simulink model "IMM_2model_turn_rate_Com"  (R2012b)
settings: Solver=FixedStepDiscrete  StartTime=0.0  StopTime=SimulStop  FixedStep=0.05  RelTol=1e-3
values from neighbouring files (symbols this model uses):
  A1 = [1 T 0 0;       0 1 0 0;       0 0 1 T;       0 0 0 1]    [parameter.m]
  A2 = [1 sin(r2*T)/r2 0 -(1-cos(r2*T))/r2;      0 cos(r2*T) 0 -sin(r2*T);      0 (1-cos(r2*T))/r2 1 sin(r2*T)/r2;      0 sin(r2*T) 0 cos(r2*T)]    [parameter.m]
  A3 = [1 T1 0 0;       0 1 0 0;       0 0 1 T1;       0 0 0 1]    [parameter.m]
  A4 = [1 sin(r2*T1)/r2 0 -(1-cos(r2*T1))/r2;      0 cos(r2*T1) 0 -sin(r2*T1);      0 (1-cos(r2*T1))/r2 1 sin(r2*T1)/r2;      0 sin(r2*T1) 0 cos(r2*T1)]    [parameter.m]
  C = [1 0 0 0; 0 0 1 0]    [parameter.m]
  mu1_init = 0.5    [parameter.m]
  mu2_init = 0.5    [parameter.m]
  P_init = eye(4)*5    [parameter.m]
  PHI = [0.99 0.01; 0.01 0.99]    [parameter.m]
  SimulStop = length(obv_traj1)*T    [parameter.m]
  T1 = 0.5    [parameter.m]
  V1 = Dw*Sv1*Dw'    [parameter.m]
  W1 = Bw*Sw1*Bw'    [parameter.m]
  W2 = Bw*Sw2*Bw'    [parameter.m]
  xhat_init = [obv_traj1(1,2);0 ;obv_traj1(1,3);0]    [parameter.m]
libraries: dspmtrx3 x10, dspinverses x2, commnoisgen2 x1
settings Model: Creator=DonghanLee  LastModifiedBy=DonghanLee

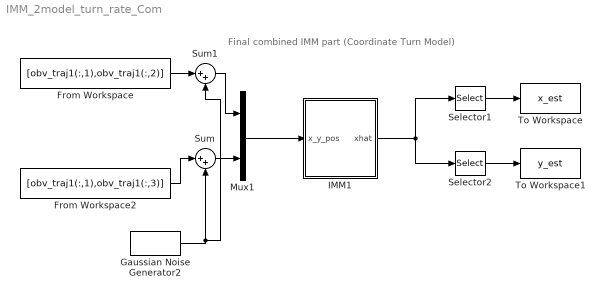
== system IMM_2model_turn_rate_Com ==
  note: Final combined IMM part (Coordinate Turn Model)
  From Workspace : FromWorkspace  VariableName=[obv_traj1(:,1),obv_traj1(:,2)]  SampleTime=0
  From Workspace2 : FromWorkspace  VariableName=[obv_traj1(:,1),obv_traj1(:,3)]  SampleTime=0
  Gaussian Noise Generator2 : commnoisgen2/Gaussian Noise Generator  m=0  d=noise  s=0  Ts=0.05  frameBased=off  sampPerFrame=1  orient=off  outDataType=double
  IMM1 : Subsystem
  Mux1 : Mux  Inputs=2
  Selector1 : Selector  InputPortWidth=4  IndexOptions=Index vector (dialog)  Indices=[1 2]  OutputSizes=1
  Selector2 : Selector  InputPortWidth=4  IndexOptions=Index vector (dialog)  Indices=[3 4]  OutputSizes=1
  Sum : Sum  Inputs=|++
  Sum1 : Sum  Inputs=|++
  To Workspace : ToWorkspace  VariableName=x_est  SampleTime=-1
  To Workspace1 : ToWorkspace  VariableName=y_est  SampleTime=-1
  wires:
  Mux1/1 -> IMM1/1(x_y_pos)
  Gaussian Noise Generator2/1 -> Sum1/2, Sum/2
  From Workspace2/1 -> Sum/1
  Sum/1 -> Mux1/2
  From Workspace/1 -> Sum1/1
  Sum1/1 -> Mux1/1
  IMM1/1(xhat) -> Selector2/1, Selector1/1
  Selector1/1 -> To Workspace/1
  Selector2/1 -> To Workspace1/1

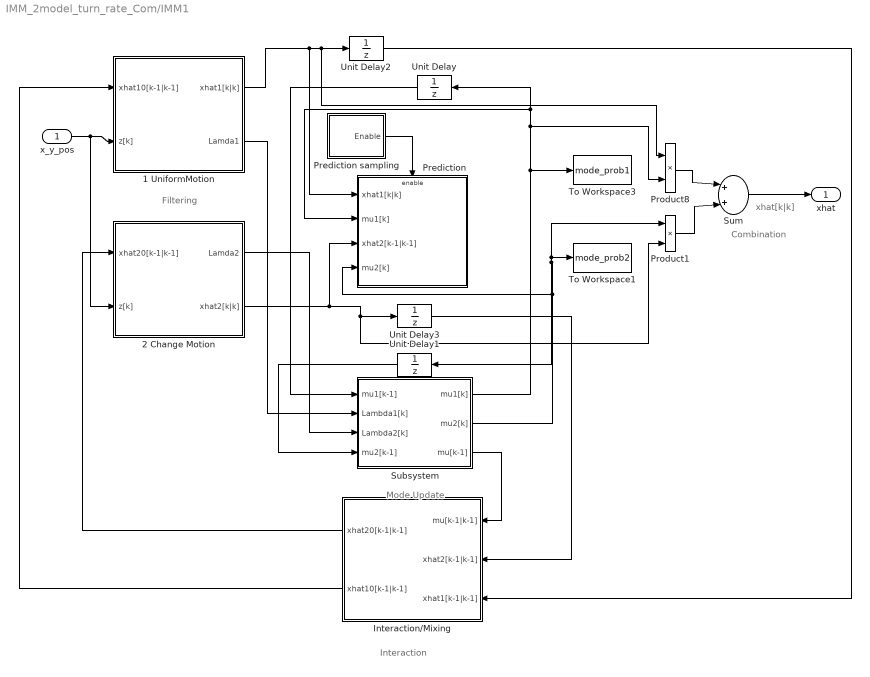
== system IMM_2model_turn_rate_Com/IMM1 ==
  note: Mode Update
  note: Interaction
  note: Filtering
  note: xhat[k|k]
  note: Combination
  x_y_pos : Inport
  "1 UniformMotion " : Subsystem
  "2 Change Motion " : Subsystem
  Interaction/Mixing : Subsystem
  Prediction : Subsystem
  Prediction sampling : Subsystem
  Product1 : Product  SaturateOnIntegerOverflow=on  OutDataTypeStr=Inherit: Same as first input
  Product8 : Product  SaturateOnIntegerOverflow=on  OutDataTypeStr=Inherit: Same as first input
  Subsystem : Subsystem
  Sum : Sum  Inputs=|++|  SaturateOnIntegerOverflow=on
  To Workspace1 : ToWorkspace  VariableName=mode_prob2  SampleTime=-1
  To Workspace3 : ToWorkspace  VariableName=mode_prob1  SampleTime=-1
  Unit Delay : UnitDelay  InitialCondition=mu1_init  SampleTime=-1
  Unit Delay1 : UnitDelay  InitialCondition=mu2_init  SampleTime=-1
  Unit Delay2 : UnitDelay  InitialCondition=xhat_init  SampleTime=-1
  Unit Delay3 : UnitDelay  InitialCondition=xhat_init  SampleTime=-1
  xhat : Outport
  wires:
  Product8/1 -> Sum/1
  Product1/1 -> Sum/2
  "2 Change Motion "/2(xhat2[k|k]) -> Prediction/3(xhat2[k-1|k-1]), Product1/2, Unit Delay3/1
  Subsystem/3(mu[k-1]) -> Interaction/Mixing/1(mu[k-1|k-1])
  Interaction/Mixing/1(xhat20[k-1|k-1]) -> "2 Change Motion "/1(xhat20[k-1|k-1])
  Interaction/Mixing/2(xhat10[k-1|k-1]) -> "1 UniformMotion "/1(xhat10[k-1|k-1])
  Sum/1 -> xhat/1
  Unit Delay/1 -> Subsystem/1(mu1[k-1])
  Unit Delay1/1 -> Subsystem/4(mu2[k-1])
  Unit Delay3/1 -> Interaction/Mixing/2(xhat2[k-1|k-1])
  Unit Delay2/1 -> Interaction/Mixing/3(xhat1[k-1|k-1])
  x_y_pos/1 -> "2 Change Motion "/2(z[k]), "1 UniformMotion "/2(z[k])
  "1 UniformMotion "/1(xhat1[k|k]) -> Prediction/1(xhat1[k|k]), Product8/1, Unit Delay2/1
  "1 UniformMotion "/2(Lamda1) -> Subsystem/2(Lambda1[k])
  "2 Change Motion "/1(Lamda2) -> Subsystem/3(Lambda2[k])
  Subsystem/1(mu1[k]) -> To Workspace3/1, Product8/2, Unit Delay/1, Prediction/2("mu1[k] ")
  Subsystem/2(mu2[k]) -> Product1/1, To Workspace1/1, Unit Delay1/1, Prediction/4(mu2[k])
  Prediction sampling/1(Enable) -> Prediction/Enable

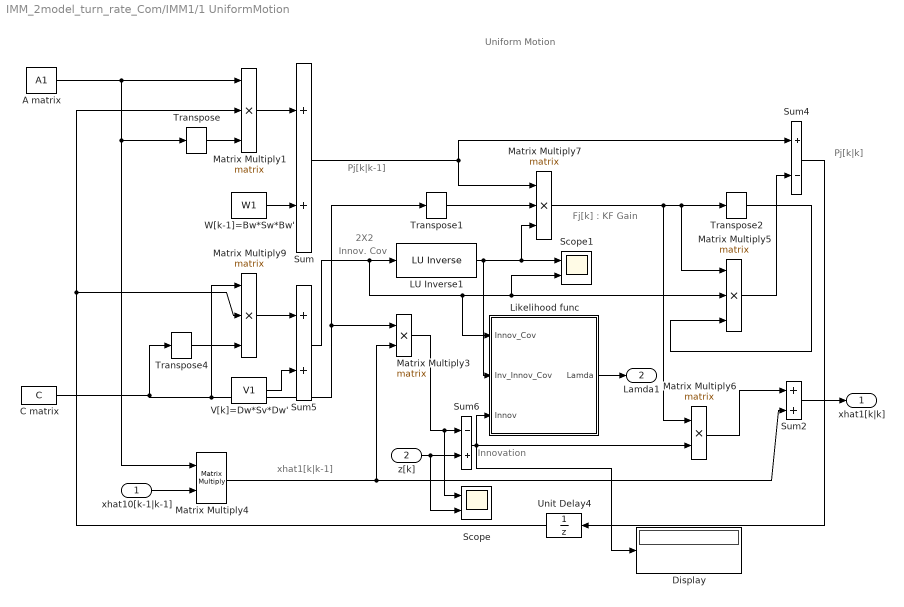
== system IMM_2model_turn_rate_Com/IMM1/1 UniformMotion  ==
  note: 2X2
  note: Pj[k|k]
  note: Innovation
  note: Innov. Cov
  note: Pj[k|k-1]
  note: xhat1[k|k-1]
  note: Uniform Motion
  note: Fj[k] : KF Gain
  xhat10[k-1|k-1] : Inport
  z[k] : Inport  Port=2
  " LU Inverse1" : dspinverses/ LU Inverse
  A matrix : Constant  Value=A1
  C matrix : Constant  Value=C
  Display : Display
  Likelihood func : Subsystem
  Matrix Multiply{1,5,7,9} (4 alike) : Product  Inputs=3  Multiplication=Matrix(*)
  Matrix Multiply3 : Product  Multiplication=Matrix(*)
  Matrix Multiply4 : Product  Multiplication=Matrix(*)
  Matrix Multiply6 : Product  Multiplication=Matrix(*)
  Scope : Scope  NumInputPorts=2
      settings: YMin=-5~5  YMax=5~20  SaveName=ScopeData10
  Scope1 : Scope  NumInputPorts=2
      settings: YMin=-0.00025~-5e+300  YMax=0.0015~3e+301  SaveName=ScopeData11
  Sum : Sum  SaturateOnIntegerOverflow=on
  Sum2 : Sum  SaturateOnIntegerOverflow=on
  Sum4 : Sum  Inputs=+-  SaturateOnIntegerOverflow=on
  Sum5 : Sum  SaturateOnIntegerOverflow=on
  Sum6 : Sum  Inputs=-+  SaturateOnIntegerOverflow=on
  Transpose{,1..2,4} (4 alike) : dspmtrx3/Transpose  Hermitian=off  overflowFlag=off
  Unit Delay4 : UnitDelay  InitialCondition=P_init  SampleTime=-1
  V[k]=Dw*Sv*Dw' : Constant  Value=V1
  "W[k-1]=Bw*Sw*Bw' " : Constant  Value=W1
  xhat1[k|k] : Outport
  Lamda1 : Outport  Port=2
  wires:
  Transpose/1 -> Matrix Multiply1/3
  A matrix/1 -> Matrix Multiply1/1, Matrix Multiply4/1, Transpose/1
  Matrix Multiply1/1 -> Sum/1
  Matrix Multiply3/1 -> Scope/1, Sum6/1
  C matrix/1 -> Transpose4/1, Matrix Multiply9/1, Transpose1/1, Matrix Multiply3/1
  Matrix Multiply4/1 -> Matrix Multiply3/2, Sum2/2
  Matrix Multiply7/1 -> Matrix Multiply6/1, Matrix Multiply5/1, Transpose2/1
  Transpose2/1 -> Matrix Multiply5/3
  Matrix Multiply6/1 -> Sum2/1
  Sum2/1 -> xhat1[k|k]/1
  "W[k-1]=Bw*Sw*Bw' "/1 -> Sum/2
  xhat10[k-1|k-1]/1 -> Matrix Multiply4/2
  Sum4/1 -> Unit Delay4/1
  Sum5/1 -> Likelihood func/1(Innov_Cov), Scope1/2, Matrix Multiply5/2, " LU Inverse1"/1
  " LU Inverse1"/1 -> Likelihood func/2(Inv_Innov_Cov), Scope1/1, Matrix Multiply7/3
  Unit Delay4/1 -> Matrix Multiply1/2, Matrix Multiply9/2
  Transpose4/1 -> Matrix Multiply9/3
  Matrix Multiply9/1 -> Sum5/1
  V[k]=Dw*Sv*Dw'/1 -> Sum5/2
  Transpose1/1 -> Matrix Multiply7/2
  z[k]/1 -> Scope/2, Sum6/2
  Sum6/1 -> Matrix Multiply6/2, Likelihood func/3(Innov), Display/1
  Matrix Multiply5/1 -> Sum4/2
  Sum/1 -> Sum4/1, Matrix Multiply7/1
  Likelihood func/1(Lamda) -> Lamda1/1

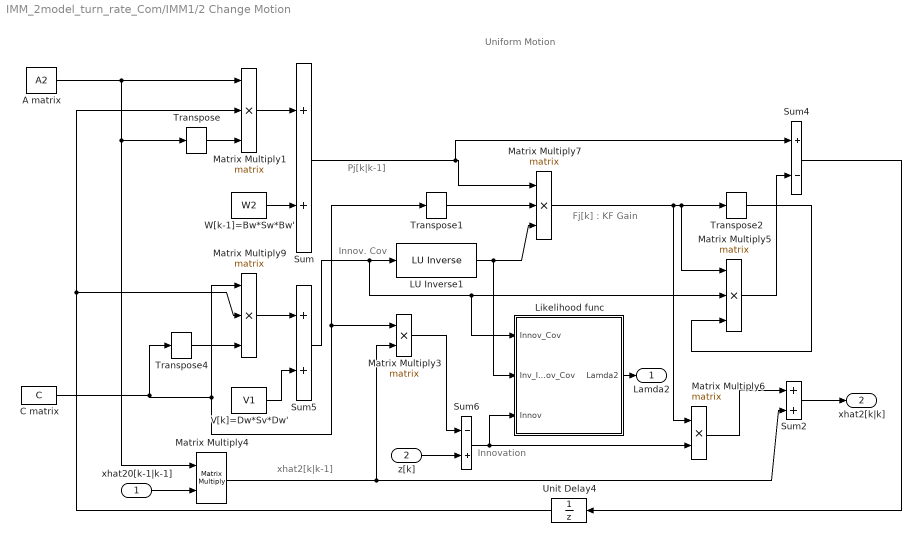
== system IMM_2model_turn_rate_Com/IMM1/2 Change Motion  ==
  note: Fj[k] : KF Gain
  note: Uniform Motion
  note: xhat2[k|k-1]
  note: Pj[k|k-1]
  note: Innov. Cov
  note: Innovation
  xhat20[k-1|k-1] : Inport
  z[k] : Inport  Port=2
  " LU Inverse1" : dspinverses/ LU Inverse
  A matrix : Constant  Value=A2
  C matrix : Constant  Value=C
  Likelihood func : Subsystem
  Matrix Multiply{1,5,7,9} (4 alike) : Product  Inputs=3  Multiplication=Matrix(*)
  Matrix Multiply3 : Product  Multiplication=Matrix(*)
  Matrix Multiply4 : Product  Multiplication=Matrix(*)
  Matrix Multiply6 : Product  Multiplication=Matrix(*)
  Sum : Sum  SaturateOnIntegerOverflow=on
  Sum2 : Sum  SaturateOnIntegerOverflow=on
  Sum4 : Sum  Inputs=+-  SaturateOnIntegerOverflow=on
  Sum5 : Sum  SaturateOnIntegerOverflow=on
  Sum6 : Sum  Inputs=-+  SaturateOnIntegerOverflow=on
  Transpose{,1..2,4} (4 alike) : dspmtrx3/Transpose  Hermitian=off  overflowFlag=off
  Unit Delay4 : UnitDelay  InitialCondition=P_init  SampleTime=-1
  V[k]=Dw*Sv*Dw' : Constant  Value=V1
  "W[k-1]=Bw*Sw*Bw' " : Constant  Value=W2
  Lamda2 : Outport
  xhat2[k|k] : Outport  Port=2
  wires:
  Sum/1 -> Matrix Multiply7/1, Sum4/1
  Matrix Multiply5/1 -> Sum4/2
  Sum6/1 -> Likelihood func/3(Innov), Matrix Multiply6/2
  z[k]/1 -> Sum6/2
  Transpose1/1 -> Matrix Multiply7/2
  V[k]=Dw*Sv*Dw'/1 -> Sum5/2
  Matrix Multiply9/1 -> Sum5/1
  Transpose4/1 -> Matrix Multiply9/3
  Unit Delay4/1 -> Matrix Multiply9/2, Matrix Multiply1/2
  " LU Inverse1"/1 -> Likelihood func/2(Inv_Innov_Cov), Matrix Multiply7/3
  Sum5/1 -> " LU Inverse1"/1, Likelihood func/1(Innov_Cov), Matrix Multiply5/2
  Sum4/1 -> Unit Delay4/1
  xhat20[k-1|k-1]/1 -> Matrix Multiply4/2
  "W[k-1]=Bw*Sw*Bw' "/1 -> Sum/2
  Sum2/1 -> xhat2[k|k]/1
  Matrix Multiply6/1 -> Sum2/1
  Transpose2/1 -> Matrix Multiply5/3
  Matrix Multiply7/1 -> Transpose2/1, Matrix Multiply5/1, Matrix Multiply6/1
  Matrix Multiply4/1 -> Sum2/2, Matrix Multiply3/2
  C matrix/1 -> Matrix Multiply3/1, Transpose1/1, Matrix Multiply9/1, Transpose4/1
  Matrix Multiply3/1 -> Sum6/1
  Matrix Multiply1/1 -> Sum/1
  A matrix/1 -> Transpose/1, Matrix Multiply4/1, Matrix Multiply1/1
  Transpose/1 -> Matrix Multiply1/3
  Likelihood func/1(Lamda2) -> Lamda2/1

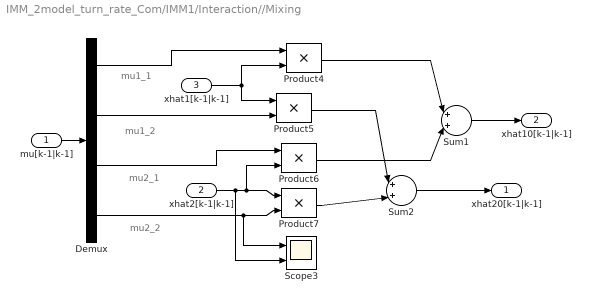
== system IMM_2model_turn_rate_Com/IMM1/Interaction//Mixing ==
  note: mu1_1
  note: mu1_2
  note: mu2_1
  note: mu2_2
  mu[k-1|k-1] : Inport
  xhat2[k-1|k-1] : Inport  Port=2
  xhat1[k-1|k-1] : Inport  Port=3
  Demux : Demux
  Product{4..7} (4 alike) : Product  SaturateOnIntegerOverflow=on  OutDataTypeStr=Inherit: Same as first input
  Scope3 : Scope  NumInputPorts=2
      settings: TimeRange=10  YMin=-5~-5  YMax=5~5  SaveName=ScopeData7
  Sum1 : Sum  Inputs=|++|  SaturateOnIntegerOverflow=on
  Sum2 : Sum  Inputs=|++|  SaturateOnIntegerOverflow=on
  xhat20[k-1|k-1] : Outport
  xhat10[k-1|k-1] : Outport  Port=2
  wires:
  Demux/2 -> Product5/2
  Demux/4 -> Scope3/1, Product7/2
  Product4/1 -> Sum1/1
  Product6/1 -> Sum1/2
  xhat1[k-1|k-1]/1 -> Product4/2, Product5/1
  Demux/1 -> Product4/1
  Demux/3 -> Product6/1
  xhat2[k-1|k-1]/1 -> Scope3/2, Product6/2, Product7/1
  Product5/1 -> Sum2/1
  Product7/1 -> Sum2/2
  Sum2/1 -> xhat20[k-1|k-1]/1
  mu[k-1|k-1]/1 -> Demux/1
  Sum1/1 -> xhat10[k-1|k-1]/1

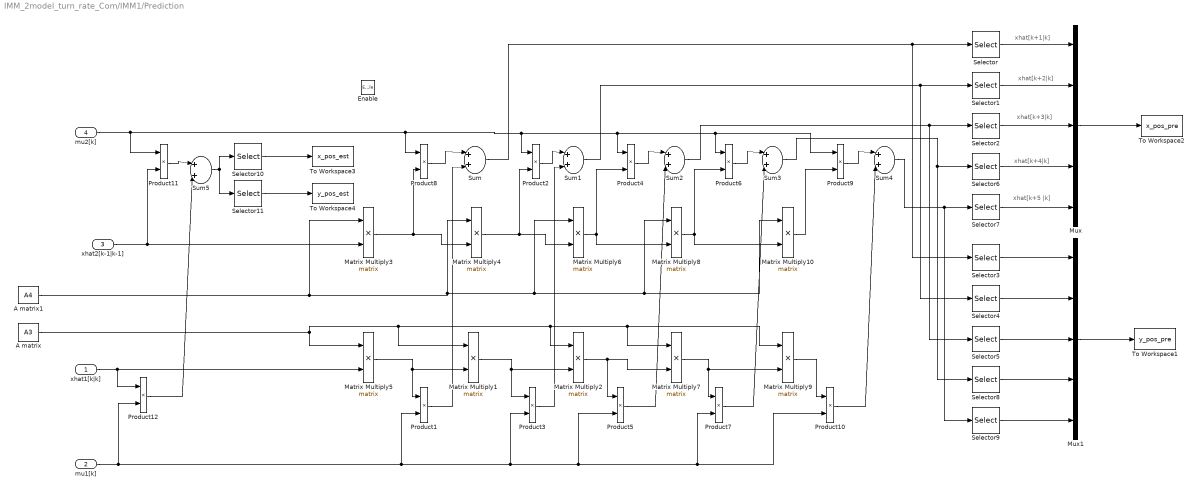
== system IMM_2model_turn_rate_Com/IMM1/Prediction ==
  note: xhat[k+4|k]
  note: xhat[k+3|k]
  note: xhat[k+1|k]
  note: xhat[k+2|k]
  note: xhat[k+5 |k]
  xhat1[k|k] : Inport
  "mu1[k] " : Inport  Port=2
  xhat2[k-1|k-1] : Inport  Port=3
  mu2[k] : Inport  Port=4
  Enable : EnablePort
  A matrix : Constant  Value=A3
  A matrix1 : Constant  Value=A4
  Matrix Multiply{1..10} (10 alike) : Product  Multiplication=Matrix(*)
  Mux : Mux  Inputs=5
  Mux1 : Mux  Inputs=5
  Product{1..12} (12 alike) : Product  SaturateOnIntegerOverflow=on  OutDataTypeStr=Inherit: Same as first input
  Selector{,1..2,6..7,10} (6 alike) : Selector  InputPortWidth=4  IndexOptions=Index vector (dialog)  Indices=[1]  OutputSizes=1
  Selector{3..5,8..9,11} (6 alike) : Selector  InputPortWidth=4  IndexOptions=Index vector (dialog)  Indices=[3]  OutputSizes=1
  Sum{,1..5} (6 alike) : Sum  Inputs=|++|  SaturateOnIntegerOverflow=on
  To Workspace1 : ToWorkspace  VariableName=y_pos_pre  SampleTime=-1
  To Workspace2 : ToWorkspace  VariableName=x_pos_pre  SampleTime=-1
  To Workspace3 : ToWorkspace  VariableName=x_pos_est  SampleTime=-1
  To Workspace4 : ToWorkspace  VariableName=y_pos_est  SampleTime=-1
  wires:
  A matrix/1 -> Matrix Multiply9/1, Matrix Multiply7/1, Matrix Multiply2/1, Matrix Multiply1/1, Matrix Multiply5/1
  xhat1[k|k]/1 -> Product12/1, Matrix Multiply5/2
  Matrix Multiply3/1 -> Product8/2, Matrix Multiply4/2
  Product1/1 -> Sum/2
  Product8/1 -> Sum/1
  Matrix Multiply4/1 -> Matrix Multiply6/2, Product2/2
  Product2/1 -> Sum1/1
  Product3/1 -> Sum1/2
  Matrix Multiply6/1 -> Matrix Multiply8/2, Product4/2
  Matrix Multiply2/1 -> Matrix Multiply7/2, Product5/1
  Product4/1 -> Sum2/1
  Product5/1 -> Sum2/2
  Mux/1 -> To Workspace2/1
  Mux1/1 -> To Workspace1/1
  Matrix Multiply5/1 -> Product1/1, Matrix Multiply1/2
  Matrix Multiply1/1 -> Product3/1, Matrix Multiply2/2
  Matrix Multiply8/1 -> Product6/2, Matrix Multiply10/2
  Matrix Multiply7/1 -> Matrix Multiply9/2, Product7/1
  Product6/1 -> Sum3/1
  Product7/1 -> Sum3/2
  mu2[k]/1 -> Product11/1, Product8/1, Product9/1, Product6/1, Product4/1, Product2/1
  "mu1[k] "/1 -> Product12/2, Product1/2, Product10/2, Product7/2, Product5/2, Product3/2
  Matrix Multiply10/1 -> Product9/2
  Matrix Multiply9/1 -> Product10/1
  Product9/1 -> Sum4/1
  Product10/1 -> Sum4/2
  Selector6/1 -> Mux/4
  Selector2/1 -> Mux/3
  Selector7/1 -> Mux/5
  Selector/1 -> Mux/1
  Selector1/1 -> Mux/2
  Selector3/1 -> Mux1/1
  Selector4/1 -> Mux1/2
  Selector5/1 -> Mux1/3
  Selector8/1 -> Mux1/4
  Selector9/1 -> Mux1/5
  Sum/1 -> Selector/1, Selector3/1
  Sum1/1 -> Selector4/1, Selector1/1
  Sum2/1 -> Selector5/1, Selector2/1
  Sum3/1 -> Selector8/1, Selector6/1
  Sum4/1 -> Selector9/1, Selector7/1
  A matrix1/1 -> Matrix Multiply3/1, Matrix Multiply6/1, Matrix Multiply8/1, Matrix Multiply10/1, Matrix Multiply4/1
  xhat2[k-1|k-1]/1 -> Product11/2, Matrix Multiply3/2
  Product11/1 -> Sum5/1
  Product12/1 -> Sum5/2
  Sum5/1 -> Selector11/1, Selector10/1
  Selector10/1 -> To Workspace3/1
  Selector11/1 -> To Workspace4/1

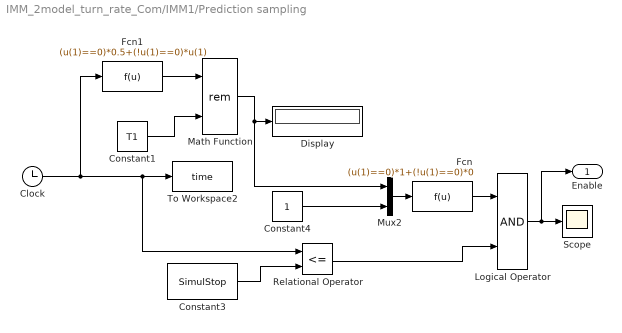
== system IMM_2model_turn_rate_Com/IMM1/Prediction sampling ==
  Clock : Clock
  Constant1 : Constant  Value=T1
  Constant3 : Constant  Value=SimulStop
  Constant4 : Constant
  Display : Display
  Fcn : Fcn  Expr=(u(1)==0)*1+(!u(1)==0)*0
  Fcn1 : Fcn  Expr=(u(1)==0)*0.5+(!u(1)==0)*u(1)
  Logical Operator : Logic  AllPortsSameDT=off  OutDataTypeStr=boolean
  Math Function : Math  Operator=rem  SaturateOnIntegerOverflow=on
  Mux2 : Mux  Inputs=2
  Relational Operator : RelationalOperator  Operator=<=  OutDataTypeStr=boolean
  Scope : Scope
      settings: SaveName=ScopeData2
  To Workspace2 : ToWorkspace  VariableName=time  SampleTime=-1
  Enable : Outport
  wires:
  Clock/1 -> Fcn1/1, Relational Operator/1, To Workspace2/1
  Constant1/1 -> Math Function/2
  Math Function/1 -> Mux2/1, Display/1
  Logical Operator/1 -> Enable/1, Scope/1
  Fcn/1 -> Logical Operator/1
  Relational Operator/1 -> Logical Operator/2
  Constant3/1 -> Relational Operator/2
  Constant4/1 -> Mux2/2
  Mux2/1 -> Fcn/1
  Fcn1/1 -> Math Function/1

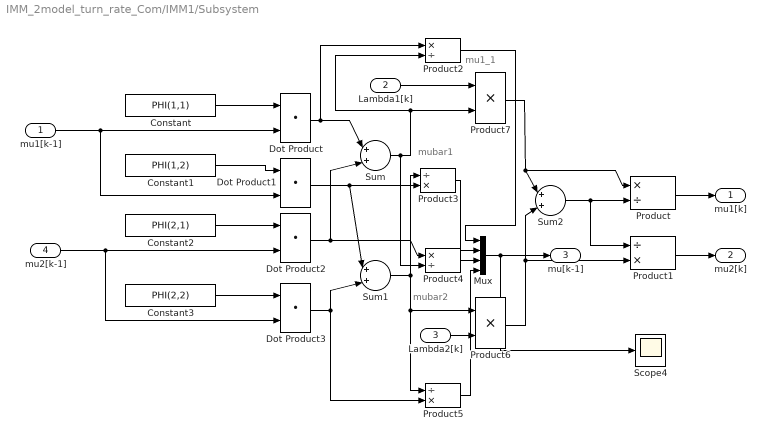
== system IMM_2model_turn_rate_Com/IMM1/Subsystem ==
  note: mubar1
  note: mubar2
  note: mu1_1
  mu1[k-1] : Inport
  Lambda1[k] : Inport  Port=2
  Lambda2[k] : Inport  Port=3
  mu2[k-1] : Inport  Port=4
  Constant : Constant  Value=PHI(1,1)
  Constant1 : Constant  Value=PHI(1,2)
  Constant2 : Constant  Value=PHI(2,1)
  Constant3 : Constant  Value=PHI(2,2)
  Dot Product{,1..3} (4 alike) : DotProduct  InputSameDT=on  OutDataTypeStr=Inherit: Inherit via internal rule
  Mux : Mux
  Product : Product  Inputs=*/  SaturateOnIntegerOverflow=on  OutDataTypeStr=Inherit: Same as first input
  Product1 : Product  Inputs=/*  SaturateOnIntegerOverflow=on  OutDataTypeStr=Inherit: Same as first input
  Product2 : Product  Inputs=*/  SaturateOnIntegerOverflow=on  OutDataTypeStr=Inherit: Same as first input
  Product3 : Product  Inputs=/*  SaturateOnIntegerOverflow=on  OutDataTypeStr=Inherit: Same as first input
  Product4 : Product  Inputs=*/  SaturateOnIntegerOverflow=on  OutDataTypeStr=Inherit: Same as first input
  Product5 : Product  Inputs=/*  SaturateOnIntegerOverflow=on  OutDataTypeStr=Inherit: Same as first input
  Product6 : Product  SaturateOnIntegerOverflow=on  OutDataTypeStr=Inherit: Same as first input
  Product7 : Product  SaturateOnIntegerOverflow=on  OutDataTypeStr=Inherit: Same as first input
  Scope4 : Scope
      settings: YMin=2.77556e-17  YMax=1  SaveName=ScopeData31
  Sum : Sum  Inputs=|++|  SaturateOnIntegerOverflow=on
  Sum1 : Sum  Inputs=|++|  SaturateOnIntegerOverflow=on
  Sum2 : Sum  Inputs=|++|  SaturateOnIntegerOverflow=on
  mu1[k] : Outport
  mu2[k] : Outport  Port=2
  mu[k-1] : Outport  Port=3
  wires:
  Constant/1 -> Dot Product/1
  Constant1/1 -> Dot Product1/1
  Constant2/1 -> Dot Product2/1
  Constant3/1 -> Dot Product3/1
  mu1[k-1]/1 -> Dot Product/2, Dot Product1/2
  mu2[k-1]/1 -> Dot Product2/2, Dot Product3/2
  Dot Product/1 -> Sum/1, Product2/1
  Dot Product2/1 -> Sum/2, Product4/1
  Dot Product1/1 -> Sum1/1, Product3/2
  Dot Product3/1 -> Sum1/2, Product5/2
  Sum1/1 -> Product5/1, Product6/1, Product3/1
  Sum/1 -> Product2/2, Product7/2, Product4/2
  Lambda1[k]/1 -> Product7/1
  Lambda2[k]/1 -> Product6/2
  Product7/1 -> Sum2/1, Product/1
  Product6/1 -> Sum2/2, Product1/2
  Sum2/1 -> Product/2, Product1/1
  Product/1 -> mu1[k]/1
  Product1/1 -> mu2[k]/1
  Product4/1 -> Mux/3
  Product2/1 -> Mux/1
  Product3/1 -> Mux/2
  Product5/1 -> Mux/4
  Mux/1 -> mu[k-1]/1, Scope4/1

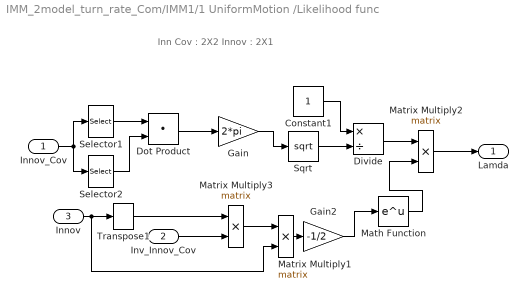
== system IMM_2model_turn_rate_Com/IMM1/1 UniformMotion /Likelihood func ==
  note: Inn Cov : 2X2
      | Innov : 2X1
  Innov_Cov : Inport
  Inv_Innov_Cov : Inport  Port=2
  Innov : Inport  Port=3
  Constant1 : Constant
  Divide : Product  Inputs=*/
  Dot Product : DotProduct  InputSameDT=on  OutDataTypeStr=Inherit: Inherit via internal rule
  Gain : Gain  Gain=2*pi
  Gain2 : Gain  Gain=-1/2
  Math Function : Math  SaturateOnIntegerOverflow=on
  Matrix Multiply1 : Product  Multiplication=Matrix(*)
  Matrix Multiply2 : Product  Multiplication=Matrix(*)
  Matrix Multiply3 : Product  Multiplication=Matrix(*)
  Selector1 : Selector  NumberOfDimensions=2  InputPortWidth=4  IndexOptions=Index vector (dialog),Index vector (dialog)  Indices=[1],[1]  OutputSizes=1,1
  Selector2 : Selector  NumberOfDimensions=2  InputPortWidth=4  IndexOptions=Index vector (dialog),Index vector (dialog)  Indices=[2],[2]  OutputSizes=1,1
  Sqrt : Sqrt  SaturateOnIntegerOverflow=on
  Transpose1 : dspmtrx3/Transpose  Hermitian=off  overflowFlag=off
  Lamda : Outport
  wires:
  Gain/1 -> Sqrt/1
  Sqrt/1 -> Divide/2
  Constant1/1 -> Divide/1
  Divide/1 -> Matrix Multiply2/1
  Math Function/1 -> Matrix Multiply2/2
  Innov/1 -> Matrix Multiply1/2, Transpose1/1
  Inv_Innov_Cov/1 -> Matrix Multiply3/2
  Transpose1/1 -> Matrix Multiply3/1
  Matrix Multiply3/1 -> Matrix Multiply1/1
  Matrix Multiply2/1 -> Lamda/1
  Matrix Multiply1/1 -> Gain2/1
  Gain2/1 -> Math Function/1
  Innov_Cov/1 -> Selector2/1, Selector1/1
  Selector2/1 -> Dot Product/2
  Selector1/1 -> Dot Product/1
  Dot Product/1 -> Gain/1

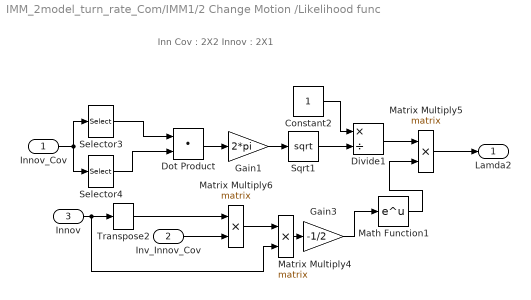
== system IMM_2model_turn_rate_Com/IMM1/2 Change Motion /Likelihood func ==
  note: Inn Cov : 2X2
      | Innov : 2X1
  Innov_Cov : Inport
  Inv_Innov_Cov : Inport  Port=2
  Innov : Inport  Port=3
  Constant2 : Constant
  Divide1 : Product  Inputs=*/
  Dot Product : DotProduct  InputSameDT=on  OutDataTypeStr=Inherit: Inherit via internal rule
  Gain1 : Gain  Gain=2*pi
  Gain3 : Gain  Gain=-1/2
  Math Function1 : Math  SaturateOnIntegerOverflow=on
  Matrix Multiply4 : Product  Multiplication=Matrix(*)
  Matrix Multiply5 : Product  Multiplication=Matrix(*)
  Matrix Multiply6 : Product  Multiplication=Matrix(*)
  Selector3 : Selector  NumberOfDimensions=2  InputPortWidth=4  IndexOptions=Index vector (dialog),Index vector (dialog)  Indices=[1],[1]  OutputSizes=1,1
  Selector4 : Selector  NumberOfDimensions=2  InputPortWidth=4  IndexOptions=Index vector (dialog),Index vector (dialog)  Indices=[2],[2]  OutputSizes=1,1
  Sqrt1 : Sqrt  SaturateOnIntegerOverflow=on
  Transpose2 : dspmtrx3/Transpose  Hermitian=off  overflowFlag=off
  Lamda2 : Outport
  wires:
  Gain1/1 -> Sqrt1/1
  Sqrt1/1 -> Divide1/2
  Constant2/1 -> Divide1/1
  Divide1/1 -> Matrix Multiply5/1
  Math Function1/1 -> Matrix Multiply5/2
  Innov/1 -> Matrix Multiply4/2, Transpose2/1
  Inv_Innov_Cov/1 -> Matrix Multiply6/2
  Transpose2/1 -> Matrix Multiply6/1
  Matrix Multiply6/1 -> Matrix Multiply4/1
  Matrix Multiply5/1 -> Lamda2/1
  Matrix Multiply4/1 -> Gain3/1
  Gain3/1 -> Math Function1/1
  Innov_Cov/1 -> Selector4/1, Selector3/1
  Selector3/1 -> Dot Product/1
  Selector4/1 -> Dot Product/2
  Dot Product/1 -> Gain1/1
